simulink model "TestPitchController"  (R2016b)
settings: Solver=VariableStepAuto  StartTime=0.0  StopTime=20  RelTol=1e-3
undefined symbols (not defined in the file): DthD, I, IthD, K_R, K_T, Pth, PthD
libraries: simulink_extras x3
settings Model: Creator=jban039  LastModifiedBy=jban039

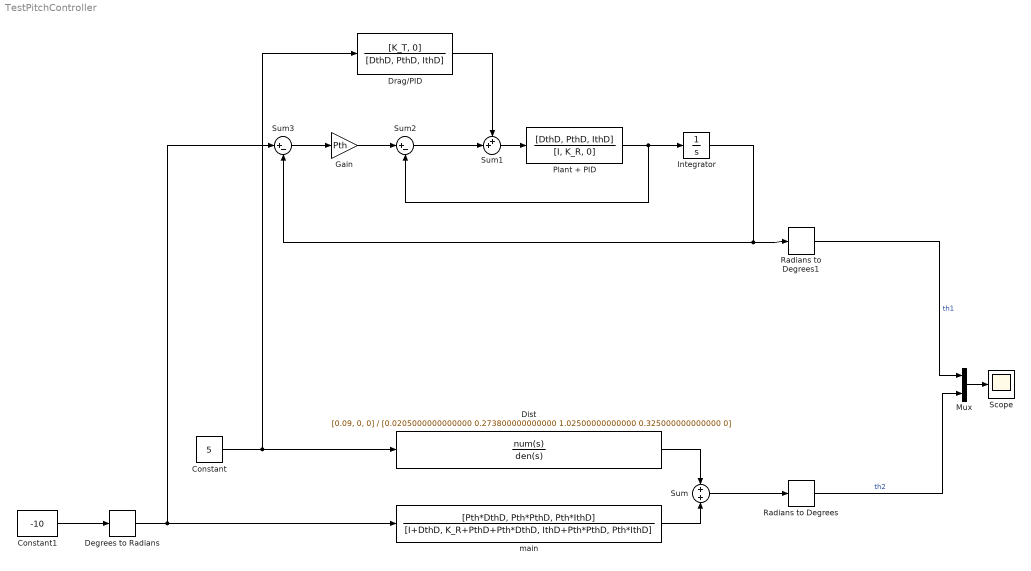
== system TestPitchController ==
  Constant : Constant  Value=5
  Constant1 : Constant  Value=-10
  Degrees to Radians : simulink_extras/Transformations/Degrees to Radians
  Dist : TransferFcn  Numerator=[0.09, 0, 0]  Denominator="[0.0205000000000000\t0.273800000000000\t1.02500000000000\t0.325000000000000\t0]"
  Drag/PID : TransferFcn  Numerator=[K_T, 0]  Denominator=[DthD, PthD, IthD]
  Gain : Gain  Gain=Pth
  Integrator : Integrator
  Mux : Mux  Inputs=2
  Plant + PID : TransferFcn  Numerator=[DthD, PthD, IthD]  Denominator=[I, K_R, 0]
  Radians to Degrees : simulink_extras/Transformations/Radians to Degrees
  Radians to Degrees1 : simulink_extras/Transformations/Radians to Degrees
  Scope : Scope
  Sum : Sum  Inputs=+|+
  Sum1 : Sum  Inputs=++|
  Sum2 : Sum  Inputs=|+-
  Sum3 : Sum  Inputs=|+-
  main : TransferFcn  Numerator=[Pth*DthD, Pth*PthD, Pth*IthD]  Denominator=[I+DthD, K_R+PthD+Pth*DthD, IthD+Pth*PthD, Pth*IthD]
  wires:
  Constant1/1 -> Degrees to Radians/1
  main/1 -> Sum/2
  Dist/1 -> Sum/1
  Sum/1 -> Radians to Degrees/1
  Radians to Degrees/1 -> Mux/2  "th2"
  Sum1/1 -> Plant + PID/1
  Drag/PID/1 -> Sum1/1
  Plant + PID/1 -> Sum2/2, Integrator/1
  Sum2/1 -> Sum1/2
  Gain/1 -> Sum2/1
  Sum3/1 -> Gain/1
  Degrees to Radians/1 -> main/1, Sum3/1
  Mux/1 -> Scope/1
  Radians to Degrees1/1 -> Mux/1  "th1"
  Integrator/1 -> Sum3/2, Radians to Degrees1/1
  Constant/1 -> Drag/PID/1, Dist/1
